simulink model "loop_shaping"  (R2015a)
settings: Solver=ode3  StartTime=0.0  StopTime=10.0  FixedStep=1/200  RelTol=1e-3
libraries: PoliArd x7
settings Model: ExtModeTrigDuration=2  Creator=GSavaia  LastModifiedBy=user
settings OptimizationCC: OptimizeModelRefInitCode=on  LifeSpan=1
settings DebuggingCC: UnderspecifiedInitializationDetection=Classic  MergeDetectMultiDrivingBlocksExec=none
settings HardwareCC: ProdLargestAtomicInteger=Long  ProdLargestAtomicFloat=Double  ProdEndianess=LittleEndian  ProdHWDeviceType=ARM Compatible->ARM Cortex
settings RTWCC: SystemTargetFile=realtime.tlc  GenerateMakefile=off  TemplateMakefile=realtime.tmf  Description=Run on Target Hardware  RTWVerbose=off
settings ERTTargetCC: CombineOutputUpdateFcns=off  ExtModeTransport=3  ExtModeMexFile=ext_serial_win32_comm_rtt  ExtModeMexArgs=0 1 9600  ERTSrcFileBannerTemplate=realtime_code_template.cgt  ERTHdrFileBannerTemplate=realtime_code_template.cgt  ERTDataSrcFileTemplate=realtime_code_template.cgt  ERTDataHdrFileTemplate=realtime_code_template.cgt  ERTCustomFileTemplate=realtime_file_process.tlc

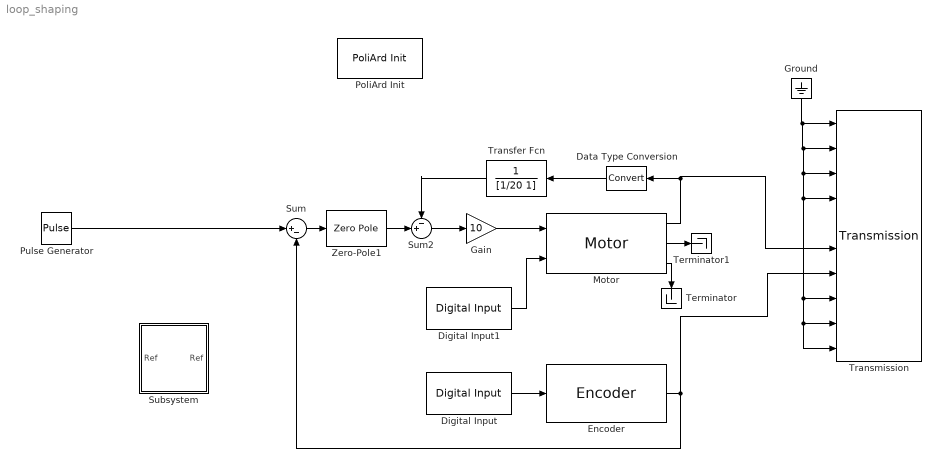
== system loop_shaping ==
  Data Type Conversion : DataTypeConversion
  Digital Input : PoliArd/Digital Input  DI_pin=2  DIsample=1/200
  Digital Input1 : PoliArd/Digital Input  DI_pin=3  DIsample=1/200
  Encoder : PoliArd/Encoder  EncoderID=1  dt_enc=-1
  Gain : Gain  Gain=10
  Ground : Ground
  Motor : PoliArd/Motor  MotorID=1  DC_bus_mask=12  dt_mot=1/200
  PoliArd Init : PoliArd/PoliArd Init
  Pulse Generator : DiscretePulseGenerator  PulseType=Time based  Amplitude=300  Period=4  PulseWidth=50  PhaseDelay=5
  Subsystem : Subsystem
  Sum : Sum  Inputs=|+-
  Sum2 : Sum  Inputs=-+|
  Terminator : Terminator
  Terminator1 : Terminator
  Transfer Fcn : TransferFcn  Denominator=[1/20 1]
  Transmission : PoliArd/Transmission  sample_freq=200  sig_to_send=6
  Zero-Pole1 : ZeroPole  Zeros=[-2+22i, -2-22i]  Poles=[0, -100]  Gain=-0.1
  wires:
  Digital Input/1 -> Encoder/1
  Gain/1 -> Motor/1
  Sum2/1 -> Gain/1
  Sum/1 -> Zero-Pole1/1
  Zero-Pole1/1 -> Sum2/2
  Motor/3 -> Terminator/1
  Motor/2 -> Terminator1/1
  Ground/1 -> Transmission/10, Transmission/9, Transmission/8, Transmission/4, Transmission/3, Transmission/2, Transmission/1
  Motor/1 -> Transmission/6, Data Type Conversion/1
  Encoder/1 -> Sum/2, Transmission/7
  Digital Input1/1 -> Motor/2
  Pulse Generator/1 -> Sum/1
  Transfer Fcn/1 -> Sum2/1
  Data Type Conversion/1 -> Transfer Fcn/1

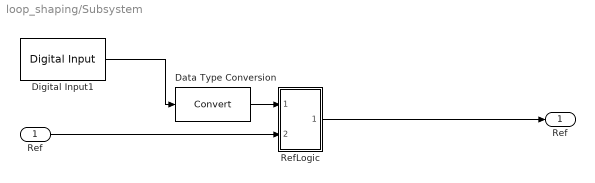
== system loop_shaping/Subsystem ==
  Ref : Inport
  Data Type Conversion : DataTypeConversion
  Digital Input1 : PoliArd/Digital Input  DI_pin=3  DIsample=1/200
  RefLogic : Subsystem
  "Ref " : Outport
  wires:
  Digital Input1/1 -> Data Type Conversion/1
  Ref/1 -> RefLogic/2(Ref)
  RefLogic/1(Out1) -> "Ref "/1
  Data Type Conversion/1 -> RefLogic/1(Enable)

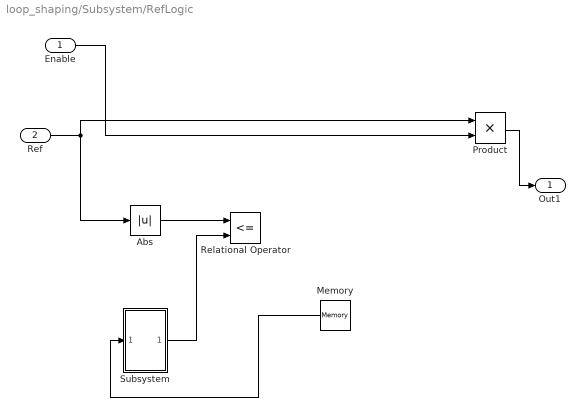
== system loop_shaping/Subsystem/RefLogic ==
  Enable : Inport
  Ref : Inport  Port=2
  Abs : Abs
  Memory : Memory
  Product : Product
  Relational Operator : RelationalOperator  Operator=<=  OutDataTypeStr=boolean
  Subsystem : Subsystem
  Out1 : Outport
  wires:
  Ref/1 -> Abs/1, Product/1
  Product/1 -> Out1/1
  ? -> Memory/1
  Subsystem/1(Out1) -> Relational Operator/2
  Enable/1 -> Product/2
  Abs/1 -> Relational Operator/1
  Memory/1 -> Subsystem/1(In1)

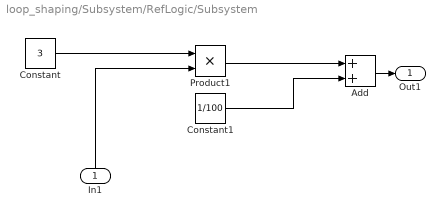
== system loop_shaping/Subsystem/RefLogic/Subsystem ==
  In1 : Inport
  Add : Sum
  Constant : Constant  Value=3
  Constant1 : Constant  Value=1/100
  Product1 : Product
  Out1 : Outport
  wires:
  Product1/1 -> Add/1
  In1/1 -> Product1/2
  Add/1 -> Out1/1
  Constant1/1 -> Add/2
  Constant/1 -> Product1/1
